simulink model "sigma_delta_fxp_hdl"  (Simulink 7.7)
settings: Solver=FixedStepDiscrete  StartTime=0.0  StopTime=.002  FixedStep=1e-7  RelTol=1e-3
libraries: simulink x1
settings Model: Creator=embed  LastModifiedBy=embed
settings SolverCC: AutoInsertRateTranBlk=on
settings OptimizationCC: BlockReduction=off  ConditionallyExecuteInputs=off

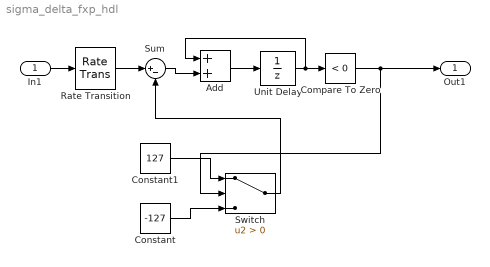
== system sigma_delta_fxp_hdl ==
  In1 : Inport  OutDataTypeStr=int8  SampleTime=512/10e6
  Add : Sum
  Compare To Zero : simulink/Logic and Bit Operations/Compare To Zero  SystemSampleTime=-1  relop=<  LogicOutDataTypeMode=boolean
  Constant : Constant  Value=-127  OutDataTypeStr=fixdt(1,16,7)
  Constant1 : Constant  Value=127  OutDataTypeStr=fixdt(1,16,7)
  Rate Transition : RateTransition  OutPortSampleTime=8/10e6
  Sum : Sum  Inputs=|+-
  Switch : Switch  Criteria=u2 > Threshold
  Unit Delay : UnitDelay  SampleTime=-1
  Out1 : Outport
  wires:
  Compare To Zero/1 -> Switch/2, Out1/1
  Rate Transition/1 -> Sum/1
  Switch/1 -> Sum/2
  Constant1/1 -> Switch/1
  Constant/1 -> Switch/3
  Unit Delay/1 -> Compare To Zero/1, Add/1
  Sum/1 -> Add/2
  Add/1 -> Unit Delay/1
  In1/1 -> Rate Transition/1
